simulink model "eTRU_prototype_2_old_perhabs_with_measurements"  (R2021b)
settings: Solver=daessc  StartTime=0.0  StopTime=5000  MaxStep=1  RelTol=1e-2  AbsTol=1e-2
PostLoadFcn:
  | eTRU_prototype_2_init
InitFcn:
  | eTRU_prototype_2_start_sim
StartFcn:
  | tic
StopFcn:
  | toc
  | PlotSimResults
values from neighbouring files (symbols this model uses):
  AirFlow = [0 0 0 0 0 0 0 0 0 0;      2205 1950 1701 1679 1297 658 0 0 0 0;      2989 2767 2610 2594 2410 2343 2274 1771 0 0;      3704 3545 3432 3422 3307 3266 3216 2958 2888 2215]    [EC_FanData.m]
  ambient_temp = 20    [eTRU_prototype_2_start_sim.m]
  asm = block.DialogPrm(1).Data    [msfcn_StaticASM.m]
  box_start_temp = 20    [eTRU_prototype_2_start_sim.m]
  cargo_start_temp = box_start_temp    (= 20)    [eTRU_prototype_2_start_sim.m]
  Power = [5 5 5 5 5 5 5 5 5 5;      185 203 227 226 229 230 231 237 239 247;      420 442 458 461 496 509 522 528 530 538;      764 811 844 846 880 892 905 969 987 989]    [EC_FanData.m]
  Pressure = LimitValue(Pressure + LimitValue(Error/dvdP, -0.1, 0.1), obj.PressureMin/100000, obj.PressureMax/100000)    [CoolPropPyWrapper.m]    (also in EC_FanData.m = [0,127,217,225,316,349,383,559,607,865])
  Speed = [0,1840,2450,3060]    [EC_FanData.m]
libraries: fl_lib x109, nesl_utility x82, simulink_extras x13, SimscapeFluids_lib x4
(part 2 of 3)

== system eTRU_prototype_2_old_perhabs_with_measurements/Evap_exv ==
  Vexp : Inport
  Gain3 : Gain  Gain=(0.007/2)^2*pi/100
  RefSensor : Subsystem
      settings: PortSchema="{\"entries\":[{\"content\":{\"sides\":[{\"content\":{\"connectorIds\":[\"LConn1\",\"Out1\"]},\"type\":\"ConnectorPlacement.EquallySpacedRectSide\",\"uuid\":\"384ca129-c08e-4242-8b56-38a57a5275bd\"},{\"content\":{\"connectorIds\":[\"RConn1\"],\"side\":\"RIGHT\"},\"type\":\"ConnectorPlacement.EquallySpacedRectSide\",\"uuid\":\"d8d27130-51db-4533-93b1-df7418a29f3a\"},{\"content\":{\"connectorIds\":[],\"side\":\"TOP\"},\"type\":\"ConnectorPlacement.EquallySpacedRectSide\",\"uuid\":\"67192aad-d15e-443e-8c24-a3a889184c8d\"},{\"content\":{\"connectorIds\":[],\"side\":\"BOTTOM\"},\"type\":\"ConnectorPlacement.EquallySpacedRectSide\",\"uuid\":\"18e5bc3a-5c8d-47f7-9803-91861ffb04f2\"}]},\"type\":\"ConnectorPlacement.EquallySpacedConnector\",\"uuid\":\"971e7a76-7cfc-4fb4-bbb6-a40c097b0bda\"}],\"packageUris\":[\"http://schema.mathworks.com/mf0/Connector/19700101\"],\"version\":\"1.0\"}"
  Simulink-PS Converter2 : nesl_utility/Simulink-PS Converter  PhysicalDomain=network_engine_domain  SubClassName=ps_input  LeftPortType=input  RightPortType=output  PseudoPeriodic=off  Frequencies=[]  NoiseDistribution=none  NoiseParameters=[]  Unit=m^2  AffineConversion=off  FilteringAndDerivatives=zero  SimscapeFilterOrder=1  InputFilterTimeConstant=0.001  UdotUserProvided=1
      settings: SourceProductBaseCode=PW,SS
  Transfer Fcn (with initial outputs) : simulink_extras/Additional Linear/Transfer Fcn (with initial outputs)  N=[1]  D="[1  1]"  Y0=0  U0=0
  Valve : fl_lib/Two-Phase Fluid/Elements/Variable Local Restriction (2P)  min_area=10e-10 mm^2  max_area=100 mm^2  area=(20/2)^2*pi mm^2  Cd=0.64  B_lam=0.999
      settings: SourceProductBaseCode=SS  InternalSimscapePortConfiguration="{\"Bottom\":[],\"Left\":[{\"id\":\"A\",\"label\":\"A\",\"type\":\"foundation.two_phase_fluid.two_phase_fluid\"},{\"id\":\"area_in\",\"label\":\"AR\",\"type\":\"input\"}],\"Right\":[{\"id\":\"B\",\"label\":\"B\",\"type\":\"foundation.two_phase_fluid.two_phase_fluid\"}],\"Top\":[]}"
  In : PMIOPort  Side=Left
  Out : PMIOPort  Port=2  Side=Right
  RefOutMeas : Outport
  wires:
  Gain3/1 -> Simulink-PS Converter2/1
  Vexp/1 -> Transfer Fcn (with initial outputs)/1
  Transfer Fcn (with initial outputs)/1 -> Gain3/1
  RefSensor/1(meas_out) -> RefOutMeas/1
  connections:
  Valve/LConn2 -- Simulink-PS Converter2/RConn1
  Valve/LConn1 -- In/RConn1
  Valve/RConn1 -- RefSensor/LConn1
  Out/RConn1 -- RefSensor/RConn1

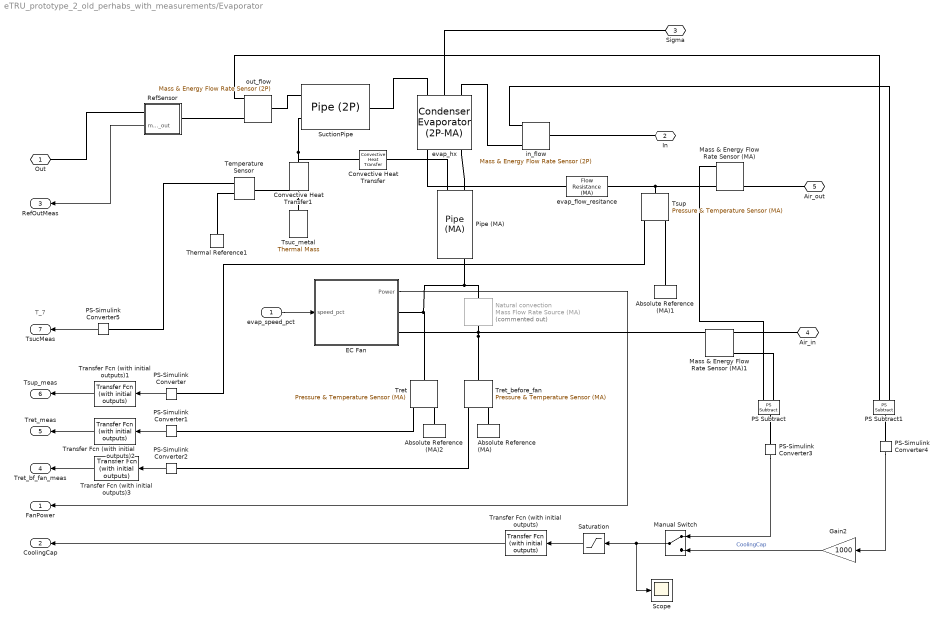
== system eTRU_prototype_2_old_perhabs_with_measurements/Evaporator ==
  note: T_7
  evap_speed_pct : Inport
  Absolute Reference (MA) : fl_lib/Moist Air/Elements/Absolute Reference (MA)
      settings: SourceProductBaseCode=SS
  Absolute Reference (MA)1 : fl_lib/Moist Air/Elements/Absolute Reference (MA)
      settings: SourceProductBaseCode=SS
  Absolute Reference (MA)2 : fl_lib/Moist Air/Elements/Absolute Reference (MA)
      settings: SourceProductBaseCode=SS
  Convective Heat Transfer : fl_lib/Thermal/Thermal Elements/Convective Heat Transfer  area=1 m^2  heat_tr_coeff=200 W/(m^2 * K)  T_specify=off  T_priority=None  T=0 K  T_nominal_specify=off  T_nominal_unit=K  T_nominal_value=1  Q_specify=off  Q_priority=None  Q=0 W  Q_nominal_specify=off  Q_nominal_unit=W  Q_nominal_value=1
  Convective Heat Transfer1 : fl_lib/Thermal/Thermal Elements/Convective Heat Transfer  area=1 m^2  heat_tr_coeff=100 W/(m^2 * K)  T_specify=off  T_priority=None  T=0 K  T_nominal_specify=off  T_nominal_unit=K  T_nominal_value=1  Q_specify=off  Q_priority=None  Q=0 W  Q_nominal_specify=off  Q_nominal_unit=W  Q_nominal_value=1
  EC Fan : Subsystem
      mask help:
      | Model of EC Fan with air flow and power consumption based on 2D table look-up.
      | Speed and pressure difference is used as table look-up input
      | The data is stored in the file EC_FanData.m that is loaded via model callback.
      | Full speed 100% is 3060 rpm
      |
      | Input:
      | Fan Speed [%] Speed reference
      | Pdiff [Pa]  pressure difference
      |
      | Output:
      | Power [Watt]Power consumption
      | Air_in, Air_out Simscape port for volumetric airflow rate
  Gain2 : Gain  Gain=1000
  Manual Switch : ManualSwitch
  Mass & Energy Flow Rate Sensor (MA) : fl_lib/Moist Air/Sensors/Mass & Energy Flow Rate Sensor (MA)
      settings: SourceProductBaseCode=SS  InternalSimscapePortConfiguration="{\"Bottom\":[],\"Left\":[{\"id\":\"A\",\"label\":\"A\",\"type\":\"foundation.moist_air.moist_air\"},{\"id\":\"Mw\",\"label\":\"Mw\",\"type\":\"output\"},{\"id\":\"Mg\",\"label\":\"Mg\",\"type\":\"output\"}],\"Right\":[{\"id\":\"B\",\"label\":\"B\",\"type\":\"foundation.moist_air.moist_air\"},{\"id\":\"M\",\"label\":\"M\",\"type\":\"output\"},{\"id\":\"PHI\",\"label\":\"Phi\",\"type\":\"output\"}],\"Top\":[]}"
  Mass & Energy Flow Rate Sensor (MA)1 : fl_lib/Moist Air/Sensors/Mass & Energy Flow Rate Sensor (MA)
      settings: SourceProductBaseCode=SS  InternalSimscapePortConfiguration="{\"Bottom\":[],\"Left\":[{\"id\":\"A\",\"label\":\"A\",\"type\":\"foundation.moist_air.moist_air\"},{\"id\":\"Mw\",\"label\":\"Mw\",\"type\":\"output\"},{\"id\":\"Mg\",\"label\":\"Mg\",\"type\":\"output\"}],\"Right\":[{\"id\":\"B\",\"label\":\"B\",\"type\":\"foundation.moist_air.moist_air\"},{\"id\":\"M\",\"label\":\"M\",\"type\":\"output\"},{\"id\":\"PHI\",\"label\":\"Phi\",\"type\":\"output\"}],\"Top\":[]}"
  Natural convection : fl_lib/Moist Air/Sources/Mass Flow Rate Source (MA)  Commented=on  power_spec=foundation.enum.power_spec.none  mass_flow=0 kg/s  area_A=1 m^2  area_B=1 m^2
      settings: SourceProductBaseCode=SS  InternalSimscapePortConfiguration="{\"Bottom\":[],\"Left\":[{\"id\":\"A\",\"label\":\"A\",\"type\":\"foundation.moist_air.moist_air\"}],\"Right\":[{\"id\":\"B\",\"label\":\"B\",\"type\":\"foundation.moist_air.moist_air\"}],\"Top\":[]}"
  PS Subtract : fl_lib/Physical Signals/Functions/PS Subtract
  PS Subtract1 : fl_lib/Physical Signals/Functions/PS Subtract
  PS-Simulink Converter{,1..5} (6 alike) : nesl_utility/PS-Simulink Converter  PhysicalDomain=network_engine_domain  SubClassName=ps_output  LeftPortType=input  RightPortType=output  PseudoPeriodic=off  Frequencies=[]  Unit=inherit  AffineConversion=off
      settings: SourceProductBaseCode=PW,SS
  Pipe (MA) : fl_lib/Moist Air/Elements/Pipe (MA)  length=1 m  area=1 m^2  Dh=1 m  length_add=0.1 m  roughness=15e-6 m  Re_lam=2000  Re_tur=4000  shape_factor=64  Nu_lam=3.66  RH_ws=1  time_constant=1e-3 s  moisture_trace_gas_source=foundation.enum.moisture_trace_gas_source.none  moisture_source_spec=foundation.enum.moisture_source_spec.vapor  moisture_mass_flow=0 kg/s  moisture_temperature_spec=foundation.enum.temperature_spec.atmospheric  moisture_temperature=293.15 K  trace_gas_mass_flow=0 kg/s  trace_gas_temperature_spec=foundation.enum.temperature_spec.atmospheric  trace_gas_temperature=293.15 K  p_I_specify=off  p_I_priority=High  p_I=0.101325 MPa  p_I_nominal_specify=off  p_I_nominal_unit=MPa  p_I_nominal_value=1  T_I_specify=off  T_I_priority=High  T_I=293.15 K  T_I_nominal_specify=off  T_I_nominal_unit=K  T_I_nominal_value=1  RH_I_specify=on  RH_I_priority=High  RH_I=0.5  RH_I_nominal_specify=off  RH_I_nominal_unit=1  RH_I_nominal_value=1  x_w_I_specify=off  x_w_I_priority=None  x_w_I=0  x_w_I_nominal_specify=off  x_w_I_nominal_unit=1  x_w_I_nominal_value=1  y_w_I_specify=off  y_w_I_priority=None  y_w_I=0  y_w_I_nominal_specify=off  y_w_I_nominal_unit=1  y_w_I_nominal_value=1  HR_I_specify=off  HR_I_priority=None  HR_I=0  HR_I_nominal_specify=off  HR_I_nominal_unit=1  HR_I_nominal_value=1  x_g_I_specify=off  x_g_I_priority=High  x_g_I=0  x_g_I_nominal_specify=off  x_g_I_nominal_unit=1  x_g_I_nominal_value=1  y_g_I_specify=off  y_g_I_priority=None  y_g_I=0  y_g_I_nominal_specify=off  y_g_I_nominal_unit=1  y_g_I_nominal_value=1
      settings: SourceProductBaseCode=SS
  RefSensor : Subsystem
  Saturation : Saturate  UpperLimit=20000  LowerLimit=-20000
  Scope : Scope
  SuctionPipe : fl_lib/Two-Phase Fluid/Elements/Pipe (2P)  length=1 m  area=0.02^2*pi m^2  Dh=0.02 m  length_add=0.1 m  roughness=15e-6 m  Re_lam=2000  Re_tur=4000  shape_factor=64  Nu_lam=3.66  inertia=simscape.enum.onoff.off  energy_spec=foundation.enum.energy_spec.quality  p_init=start_pressure_low bar  T_init=box_start_temp degC  x_init=1  alpha_init=0.1  h_init=1500 kJ/kg  u_init=1500 kJ/kg  mdot_init=0 kg/s  time_constant=0.1 s
      settings: SourceProductBaseCode=SS  InternalSimscapePortConfiguration="{\"Bottom\":[],\"Left\":[{\"id\":\"A\",\"label\":\"A\",\"type\":\"foundation.two_phase_fluid.two_phase_fluid\"},{\"id\":\"H\",\"label\":\"H\",\"type\":\"foundation.thermal.thermal\"}],\"Right\":[{\"id\":\"B\",\"label\":\"B\",\"type\":\"foundation.two_phase_fluid.two_phase_fluid\"}],\"Top\":[]}"
  Temperature Sensor : fl_lib/Thermal/Thermal Sensors/Temperature Sensor
  Thermal Reference1 : fl_lib/Thermal/Thermal Elements/Thermal Reference
  Transfer Fcn (with initial outputs) : simulink_extras/Additional Linear/Transfer Fcn (with initial outputs)  N=[0.1]  D=[1 0.1]  Y0=0  U0=0
  Transfer Fcn (with initial outputs)1 : simulink_extras/Additional Linear/Transfer Fcn (with initial outputs)  N=[0.1]  D="[1  0.1]"  Y0=box_start_temp+273.15  U0=box_start_temp+273.15
  Transfer Fcn (with initial outputs)2 : simulink_extras/Additional Linear/Transfer Fcn (with initial outputs)  N=[0.1]  D="[1  0.1]"  Y0=box_start_temp+273.15  U0=box_start_temp+273.15
  Transfer Fcn (with initial outputs)3 : simulink_extras/Additional Linear/Transfer Fcn (with initial outputs)  N=[0.1]  D="[1  0.1]"  Y0=box_start_temp+273.15  U0=box_start_temp+273.15
  Tret : fl_lib/Moist Air/Sensors/Pressure & Temperature Sensor (MA)
      settings: SourceProductBaseCode=SS  InternalSimscapePortConfiguration="{\"Bottom\":[],\"Left\":[{\"id\":\"A\",\"label\":\"A\",\"type\":\"foundation.moist_air.moist_air\"}],\"Right\":[{\"id\":\"B\",\"label\":\"B\",\"type\":\"foundation.moist_air.moist_air\"},{\"id\":\"P\",\"label\":\"P\",\"type\":\"output\"},{\"id\":\"T\",\"label\":\"T\",\"type\":\"output\"}],\"Top\":[]}"
  Tret_before_fan : fl_lib/Moist Air/Sensors/Pressure & Temperature Sensor (MA)
      settings: SourceProductBaseCode=SS  InternalSimscapePortConfiguration="{\"Bottom\":[],\"Left\":[{\"id\":\"A\",\"label\":\"A\",\"type\":\"foundation.moist_air.moist_air\"}],\"Right\":[{\"id\":\"B\",\"label\":\"B\",\"type\":\"foundation.moist_air.moist_air\"},{\"id\":\"P\",\"label\":\"P\",\"type\":\"output\"},{\"id\":\"T\",\"label\":\"T\",\"type\":\"output\"}],\"Top\":[]}"
  Tsuc_metal : fl_lib/Thermal/Thermal Elements/Thermal Mass  mass=0.5 kg  sp_heat=900 J/kg/K  T_specify=on  T_priority=None  T=box_start_temp degC  T_nominal_specify=off  T_nominal_unit=K  T_nominal_value=1  Q_specify=off  Q_priority=None  Q=0 W  Q_nominal_specify=off  Q_nominal_unit=W  Q_nominal_value=1
  Tsup : fl_lib/Moist Air/Sensors/Pressure & Temperature Sensor (MA)
      settings: SourceProductBaseCode=SS  InternalSimscapePortConfiguration="{\"Bottom\":[],\"Left\":[{\"id\":\"A\",\"label\":\"A\",\"type\":\"foundation.moist_air.moist_air\"}],\"Right\":[{\"id\":\"B\",\"label\":\"B\",\"type\":\"foundation.moist_air.moist_air\"},{\"id\":\"P\",\"label\":\"P\",\"type\":\"output\"},{\"id\":\"T\",\"label\":\"T\",\"type\":\"output\"}],\"Top\":[]}"
  evap_flow_resitance : fl_lib/Moist Air/Elements/Flow Resistance (MA)  delta_p_nominal=250 Pa  mdot_nominal=1 kg/s  rho_nominal=0 kg/m^3  area=1 m^2  laminar_fraction=1e-3
      settings: SourceProductBaseCode=SS
  evap_hx : SimscapeFluids_lib/Fluid Network Interfaces/Heat Exchangers/Condenser Evaporator (2P-MA)  flow_arrangement=fluids.interfaces.heat_exchangers.enum.FlowArrangement2PMA.Counter  cross_flow_arrangement=fluids.interfaces.heat_exchangers.enum.CrossFlowArrangement2PMA.UnmixedUnmixed  R_wall=0.1 K/kW  area_A1=0.02 m^2  area_B1=0.02 m^2  area_A2=1 m^2  area_B2=1 m^2  tube_num_2P=14  tube_length_2P=1.8*6 m  tube_cross_section_2P=fluids.interfaces.heat_exchangers.enum.TubeCrossSection.Circular  tube_diameter_2P=0.01 m  tube_width_2P=0.1 m  tube_height_2P=0.1 m  tube_inner_diameter_2P=0.05 m  tube_outer_diameter_2P=0.1 m  tube_flow_area_2P=0.01 m^2  tube_wetted_perimeter_2P=0.4 m  tube_heat_perimeter_2P=0.4 m  tube_pressure_loss_spec_2P=fluids.interfaces.heat_exchangers.enum.TubePressureLossSpec2P.Haaland  tube_loss_coeff_2P=10  tube_length_add_2P=0.5 m  tube_roughness_pressure_2P=0.001 m  tube_Re_lam_pressure_2P=2000  tube_Re_tur_pressure_2P=4000  tube_shape_factor_generic_2P=64  tube_heat_coeff_spec_2P=fluids.interfaces.heat_exchangers.enum.TubeHeatCoeffSpec2P.Colburn  tube_colburn_coeff_liq_2P=[.023, .8, .33]  tube_colburn_coeff_mix_2P=[.05, .8, .33]  tube_colburn_coeff_vap_2P=[.023, .8, .33]  tube_roughness_heat_2P=15e-6 m  tube_Re_lam_heat_2P=2000  tube_Re_tur_heat_2P=4000  tube_Nu_lam_generic_2P=3.66  fouling_factor_2P=0.1 K*m^2/kW  fin_area_2P=0.1 m^2  fin_efficiency_2P=0.5  energy_spec_2P=foundation.enum.energy_spec.quality  p_init_2P=start_pressure_low bar  T_init_2P=box_start_temp degC  x_init_2P=0.7  alpha_init_2P=0.5  h_init_2P=1500 kJ/kg  u_init_2P=1500 kJ/kg  flow_geometry_MA=fluids.interfaces.heat_exchangers.enum.FlowGeometryMA.AcrossTubeBank  tube_num_MA=1  tube_length_MA=5 m  tube_cross_section_MA=fluids.interfaces.heat_exchangers.enum.TubeCrossSection.Circular  tube_diameter_MA=0.1 m  tube_width_MA=0.1 m  tube_height_MA=0.1 m  tube_inner_diameter_MA=0.05 m  tube_outer_diameter_MA=0.1 m  tube_flow_area_MA=0.01 m^2  tube_wetted_perimeter_MA=0.4 m  tube_heat_perimeter_MA=0.4 m  tube_pressure_loss_spec_MA=fluids.interfaces.heat_exchangers.enum.TubePressureLossSpec.Haaland  tube_loss_coeff_MA=1  tube_length_add_MA=0.1 m  tube_roughness_pressure_MA=15e-6 m  tube_Re_lam_pressure_MA=2000  tube_Re_tur_pressure_MA=4000  tube_shape_factor_generic_MA=64  tube_heat_coeff_spec_MA=fluids.interfaces.heat_exchangers.enum.TubeHeatCoeffSpec.Gneilinski  tube_colburn_coeff_MA=[0.23, 0.8, 1 / 3]  tube_roughness_heat_MA=15e-6 m  tube_Re_lam_heat_MA=2000  tube_Re_tur_heat_MA=4000  tube_Nu_lam_generic_MA=3.66  bank_arrangement_MA=fluids.interfaces.heat_exchangers.enum.BankArrangement.Staggered  bank_num_rows_MA=6  bank_tubes_per_row_MA=14  bank_width_MA=0.3 m  bank_tube_diameter_MA=0.012 m  bank_longitudinal_pitch_MA=0.04 m  bank_transverse_pitch_MA=0.04 m  bank_pressure_loss_spec_MA=fluids.interfaces.heat_exchangers.enum.BankPressureLossSpec.Euler  bank_euler_MA=1  bank_heat_coeff_spec_MA=fluids.interfaces.heat_exchangers.enum.BankHeatCoeffSpec.Martin  bank_colburn_coeff_MA=[.27, .63, .36]  generic_flow_area_MA=0.1 m^2  generic_heat_area_MA=2 m^2  generic_volume_MA=1 m^3  generic_loss_coeff_MA=1  generic_colburn_coeff_MA=[0.23, 0.8, 1 / 3]  fouling_factor_MA=0.1 K*m^2/kW  fin_area_MA=50 m^2  fin_efficiency_MA=0.8  p_init_MA=0.101325 MPa  T_init_MA=box_start_temp degC  moisture_spec_MA=foundation.enum.moisture_spec.mole_fraction  RH_init_MA=0.5  x_w_init_MA=0.01  y_w_init_MA=0.01  HR_init_MA=0.01  trace_gas_spec_MA=foundation.enum.trace_gas_spec.mole_fraction  x_g_init_MA=0.001  y_g_init_MA=0.001  RH_ws_MA=1
      settings: SourceProductBaseCode=SH  InternalSimscapePortConfiguration="{\"Bottom\":[],\"Left\":[{\"id\":\"A1\",\"label\":\"A1\",\"type\":\"foundation.two_phase_fluid.two_phase_fluid\"},{\"id\":\"Z\",\"label\":\"Z\",\"type\":\"output\"},{\"id\":\"B1\",\"label\":\"B1\",\"type\":\"foundation.two_phase_fluid.two_phase_fluid\"}],\"Right\":[{\"id\":\"A2\",\"label\":\"A2\",\"type\":\"foundation.moist_air.moist_air\"},{\"id\":\"W\",\"label\":\"W\",\"type\":\"output\"},{\"id\":\"B2\",\"label\":\"B2\",\"type\":\"foundation.moist_air.moist_air\"}],\"Top\":[]}"
  in_flow : fl_lib/Two-Phase Fluid/Sensors/Mass & Energy Flow Rate Sensor (2P)
      settings: SourceProductBaseCode=SS  InternalSimscapePortConfiguration="{\"Bottom\":[],\"Left\":[{\"id\":\"A\",\"label\":\"A\",\"type\":\"foundation.two_phase_fluid.two_phase_fluid\"}],\"Right\":[{\"id\":\"B\",\"label\":\"B\",\"type\":\"foundation.two_phase_fluid.two_phase_fluid\"},{\"id\":\"M\",\"label\":\"M\",\"type\":\"output\"},{\"id\":\"PHI\",\"label\":\"Phi\",\"type\":\"output\"}],\"Top\":[]}"
  out_flow : fl_lib/Two-Phase Fluid/Sensors/Mass & Energy Flow Rate Sensor (2P)
      settings: SourceProductBaseCode=SS  InternalSimscapePortConfiguration="{\"Bottom\":[],\"Left\":[{\"id\":\"A\",\"label\":\"A\",\"type\":\"foundation.two_phase_fluid.two_phase_fluid\"}],\"Right\":[{\"id\":\"B\",\"label\":\"B\",\"type\":\"foundation.two_phase_fluid.two_phase_fluid\"},{\"id\":\"M\",\"label\":\"M\",\"type\":\"output\"},{\"id\":\"PHI\",\"label\":\"Phi\",\"type\":\"output\"}],\"Top\":[]}"
  Out : PMIOPort  Side=Left
  In : PMIOPort  Port=2  Side=Right
  Sigma : PMIOPort  Port=3  Side=Right
  Air_in : PMIOPort  Port=4  Side=Right
  Air_out : PMIOPort  Port=5  Side=Right
  FanPower : Outport
  CoolingCap : Outport  Port=2
  RefOutMeas : Outport  Port=3
  Tret_bf_fan_meas : Outport  Port=4
  Tret_meas : Outport  Port=5
  Tsup_meas : Outport  Port=6
  TsucMeas : Outport  Port=7
  wires:
  PS-Simulink Converter/1 -> Transfer Fcn (with initial outputs)1/1
  PS-Simulink Converter1/1 -> Transfer Fcn (with initial outputs)2/1
  PS-Simulink Converter2/1 -> Transfer Fcn (with initial outputs)3/1
  Transfer Fcn (with initial outputs)1/1 -> Tsup_meas/1
  Transfer Fcn (with initial outputs)3/1 -> Tret_bf_fan_meas/1
  Transfer Fcn (with initial outputs)2/1 -> Tret_meas/1
  evap_speed_pct/1 -> EC Fan/1(speed_pct)
  EC Fan/1(Power) -> FanPower/1
  Saturation/1 -> Transfer Fcn (with initial outputs)/1
  Transfer Fcn (with initial outputs)/1 -> CoolingCap/1
  Manual Switch/1 -> Scope/1, Saturation/1
  PS-Simulink Converter3/1 -> Manual Switch/1
  PS-Simulink Converter4/1 -> Gain2/1
  Gain2/1 -> Manual Switch/2  "CoolingCap"
  PS-Simulink Converter5/1 -> TsucMeas/1
  RefSensor/1(meas_out) -> RefOutMeas/1
  connections:
  Temperature Sensor/LConn1 -- Convective Heat Transfer1/RConn1 -- Tsuc_metal/LConn1
  Thermal Reference1/LConn1 -- Temperature Sensor/RConn1
  Temperature Sensor/RConn2 -- PS-Simulink Converter5/LConn1
  Tret_before_fan/LConn1 -- EC Fan/RConn2 -- Mass & Energy Flow Rate Sensor (MA)1/LConn1 -- Natural convection/LConn1
  evap_flow_resitance/RConn1 -- Mass & Energy Flow Rate Sensor (MA)/RConn1 -- Tsup/LConn1
  Absolute Reference (MA)1/LConn1 -- Tsup/RConn1
  Absolute Reference (MA)2/LConn1 -- Tret/RConn1
  EC Fan/RConn1 -- Pipe (MA)/RConn1 -- Natural convection/RConn1 -- Tret/LConn1
  Absolute Reference (MA)/LConn1 -- Tret_before_fan/RConn1
  Tsup/RConn3 -- PS-Simulink Converter/LConn1
  Tret/RConn3 -- PS-Simulink Converter1/LConn1
  Tret_before_fan/RConn3 -- PS-Simulink Converter2/LConn1
  evap_hx/LConn3 -- SuctionPipe/RConn1
  Sigma/RConn1 -- evap_hx/LConn2
  PS-Simulink Converter3/LConn1 -- PS Subtract/RConn1
  Mass & Energy Flow Rate Sensor (MA)1/RConn1 -- Air_in/RConn1
  Mass & Energy Flow Rate Sensor (MA)/LConn1 -- Air_out/RConn1
  Mass & Energy Flow Rate Sensor (MA)/RConn3 -- PS Subtract/LConn1
  Mass & Energy Flow Rate Sensor (MA)1/RConn3 -- PS Subtract/LConn2
  in_flow/RConn3 -- PS Subtract1/LConn2
  PS Subtract1/RConn1 -- PS-Simulink Converter4/LConn1
  out_flow/RConn3 -- PS Subtract1/LConn1
  out_flow/LConn1 -- SuctionPipe/LConn1
  evap_hx/LConn1 -- in_flow/RConn1
  In/RConn1 -- in_flow/LConn1
  RefSensor/LConn1 -- out_flow/RConn1
  Out/RConn1 -- RefSensor/RConn1
  Convective Heat Transfer/RConn1 -- Pipe (MA)/LConn2
  Convective Heat Transfer1/LConn1 -- SuctionPipe/LConn2 -- Convective Heat Transfer/LConn1
  Pipe (MA)/LConn1 -- evap_hx/RConn1
  evap_flow_resitance/LConn1 -- evap_hx/RConn3

== system eTRU_prototype_2_old_perhabs_with_measurements/FT_exv ==
  VFT : Inport
  Gain2 : Gain  Gain=(0.005/2)^2*pi/100*8
  RefSensor : Subsystem
      settings: PortSchema="{\"entries\":[{\"content\":{\"sides\":[{\"content\":{\"connectorIds\":[\"LConn1\"]},\"type\":\"ConnectorPlacement.EquallySpacedRectSide\",\"uuid\":\"384ca129-c08e-4242-8b56-38a57a5275bd\"},{\"content\":{\"connectorIds\":[\"RConn1\",\"Out1\"],\"side\":\"RIGHT\"},\"type\":\"ConnectorPlacement.EquallySpacedRectSide\",\"uuid\":\"d8d27130-51db-4533-93b1-df7418a29f3a\"},{\"content\":{\"connectorIds\":[],\"side\":\"TOP\"},\"type\":\"ConnectorPlacement.EquallySpacedRectSide\",\"uuid\":\"67192aad-d15e-443e-8c24-a3a889184c8d\"},{\"content\":{\"connectorIds\":[],\"side\":\"BOTTOM\"},\"type\":\"ConnectorPlacement.EquallySpacedRectSide\",\"uuid\":\"18e5bc3a-5c8d-47f7-9803-91861ffb04f2\"}]},\"type\":\"ConnectorPlacement.EquallySpacedConnector\",\"uuid\":\"971e7a76-7cfc-4fb4-bbb6-a40c097b0bda\"}],\"packageUris\":[\"http://schema.mathworks.com/mf0/Connector/19700101\"],\"version\":\"1.0\"}"
  Simulink-PS Converter3 : nesl_utility/Simulink-PS Converter  PhysicalDomain=network_engine_domain  SubClassName=ps_input  LeftPortType=input  RightPortType=output  PseudoPeriodic=off  Frequencies=[]  NoiseDistribution=none  NoiseParameters=[]  Unit=m^2  AffineConversion=off  FilteringAndDerivatives=zero  SimscapeFilterOrder=1  InputFilterTimeConstant=0.001  UdotUserProvided=1
      settings: SourceProductBaseCode=PW,SS
  Transfer Fcn (with initial outputs)1 : simulink_extras/Additional Linear/Transfer Fcn (with initial outputs)  N=[1]  D="[1  1]"  Y0=0  U0=0
  Valve : fl_lib/Two-Phase Fluid/Elements/Variable Local Restriction (2P)  min_area=10e-10 mm^2  max_area=100 mm^2  area=(20/2)^2*pi mm^2  Cd=0.64  B_lam=0.999
      settings: SourceProductBaseCode=SS  InternalSimscapePortConfiguration="{\"Bottom\":[],\"Left\":[{\"id\":\"A\",\"label\":\"A\",\"type\":\"foundation.two_phase_fluid.two_phase_fluid\"},{\"id\":\"area_in\",\"label\":\"AR\",\"type\":\"input\"}],\"Right\":[{\"id\":\"B\",\"label\":\"B\",\"type\":\"foundation.two_phase_fluid.two_phase_fluid\"}],\"Top\":[]}"
  In : PMIOPort  Side=Left
  Out : PMIOPort  Port=2  Side=Right
  RefOutMeas : Outport
  wires:
  VFT/1 -> Transfer Fcn (with initial outputs)1/1
  Gain2/1 -> Simulink-PS Converter3/1
  Transfer Fcn (with initial outputs)1/1 -> Gain2/1
  RefSensor/1(meas_out) -> RefOutMeas/1
  connections:
  Simulink-PS Converter3/RConn1 -- Valve/LConn2
  Valve/LConn1 -- In/RConn1
  Valve/RConn1 -- RefSensor/LConn1
  Out/RConn1 -- RefSensor/RConn1

== system eTRU_prototype_2_old_perhabs_with_measurements/Flash tank ==
  Cap (2P) : fl_lib/Two-Phase Fluid/Elements/Cap (2P)  p_specify=off  p_priority=None  p=0.101325 MPa  p_nominal_specify=off  p_nominal_unit=MPa  p_nominal_value=1  u_specify=off  u_priority=None  u=1.5e+3 kJ/kg  u_nominal_specify=off  u_nominal_unit=kJ/kg  u_nominal_value=1
      settings: SourceProductBaseCode=SS  InternalSimscapePortConfiguration="{\"Bottom\":[],\"Left\":[{\"id\":\"A\",\"label\":\"\",\"type\":\"foundation.two_phase_fluid.two_phase_fluid\"}],\"Right\":[],\"Top\":[]}"
  "FT heat transfer " : fl_lib/Thermal/Thermal Elements/Convective Heat Transfer  area=0.5 m^2  heat_tr_coeff=100 W/(m^2 * K)  T_specify=off  T_priority=None  T=0 K  T_nominal_specify=off  T_nominal_unit=K  T_nominal_value=1  Q_specify=off  Q_priority=None  Q=0 W  Q_nominal_specify=off  Q_nominal_unit=W  Q_nominal_value=1
  RefSensor : Subsystem
      settings: PortSchema="{\"entries\":[{\"content\":{\"sides\":[{\"content\":{\"connectorIds\":[\"LConn1\"]},\"type\":\"ConnectorPlacement.EquallySpacedRectSide\",\"uuid\":\"384ca129-c08e-4242-8b56-38a57a5275bd\"},{\"content\":{\"connectorIds\":[\"RConn1\",\"Out1\"],\"side\":\"RIGHT\"},\"type\":\"ConnectorPlacement.EquallySpacedRectSide\",\"uuid\":\"d8d27130-51db-4533-93b1-df7418a29f3a\"},{\"content\":{\"connectorIds\":[],\"side\":\"TOP\"},\"type\":\"ConnectorPlacement.EquallySpacedRectSide\",\"uuid\":\"67192aad-d15e-443e-8c24-a3a889184c8d\"},{\"content\":{\"connectorIds\":[],\"side\":\"BOTTOM\"},\"type\":\"ConnectorPlacement.EquallySpacedRectSide\",\"uuid\":\"18e5bc3a-5c8d-47f7-9803-91861ffb04f2\"}]},\"type\":\"ConnectorPlacement.EquallySpacedConnector\",\"uuid\":\"971e7a76-7cfc-4fb4-bbb6-a40c097b0bda\"}],\"packageUris\":[\"http://schema.mathworks.com/mf0/Connector/19700101\"],\"version\":\"1.0\"}"
  RefSensor1 : Subsystem
  Tank : SimscapeFluids_lib/Two-Phase Fluid/Tanks & Accumulators/Receiver Accumulator (2P)  volume=0.005 m^3  area_AV=0.01 m^2  area_BV=0.01 m^2  area_AL=0.01 m^2  area_BL=0.01 m^2  V_frac_error=simscape.enum.assert.action.warn  V_frac_min=0.05  V_frac_max=0.95  V_frac_smooth=0.05  p_crit_error=simscape.enum.assert.action.warn  hc_vap=20 W/(m^2*K)  hc_liq=100 W/(m^2*K)  surface_area=1 m^2  receiver_accumulator_energy_spec=fluids.two_phase_fluid.enum.receiver_accumulator_energy_spec.volume_fraction  p_init=start_pressure_im bar  T_init=im_start_temp degC  M_frac_init=0.5  V_frac_init=0.5  h_init=1500 kJ/kg  u_init=1500 kJ/kg  tau_vap_cond=0.1 s
      settings: SourceProductBaseCode=SH  InternalSimscapePortConfiguration="{\"Bottom\":[],\"Left\":[{\"id\":\"AV\",\"label\":\"AV\",\"type\":\"foundation.two_phase_fluid.two_phase_fluid\"},{\"id\":\"AL\",\"label\":\"AL\",\"type\":\"foundation.two_phase_fluid.two_phase_fluid\"},{\"id\":\"H\",\"label\":\"H\",\"type\":\"foundation.thermal.thermal\"}],\"Right\":[{\"id\":\"BV\",\"label\":\"BV\",\"type\":\"foundation.two_phase_fluid.two_phase_fluid\"},{\"id\":\"BL\",\"label\":\"BL\",\"type\":\"foundation.two_phase_fluid.two_phase_fluid\"},{\"id\":\"L\",\"label\":\"L\",\"type\":\"output\"}],\"Top\":[]}"
  Liquid in : PMIOPort  Side=Left
  Vapor out : PMIOPort  Port=2  Side=Left
  Liquid out : PMIOPort  Port=3  Side=Left
  Level : PMIOPort  Port=4  Side=Right
  H : PMIOPort  Port=5  Side=Right
  liq_out_meas : Outport
  vap_out_meas : Outport  Port=2
  wires:
  RefSensor/1(meas_out) -> vap_out_meas/1
  RefSensor1/1(meas_out) -> liq_out_meas/1
  connections:
  Liquid in/RConn1 -- Tank/LConn1
  H/RConn1 -- "FT heat transfer "/RConn1
  Tank/LConn2 -- Cap (2P)/LConn1
  Tank/RConn3 -- Level/RConn1
  "FT heat transfer "/LConn1 -- Tank/LConn3
  Tank/RConn1 -- RefSensor/LConn1
  RefSensor/RConn1 -- Vapor out/RConn1
  Tank/RConn2 -- RefSensor1/LConn1
  RefSensor1/RConn1 -- Liquid out/RConn1

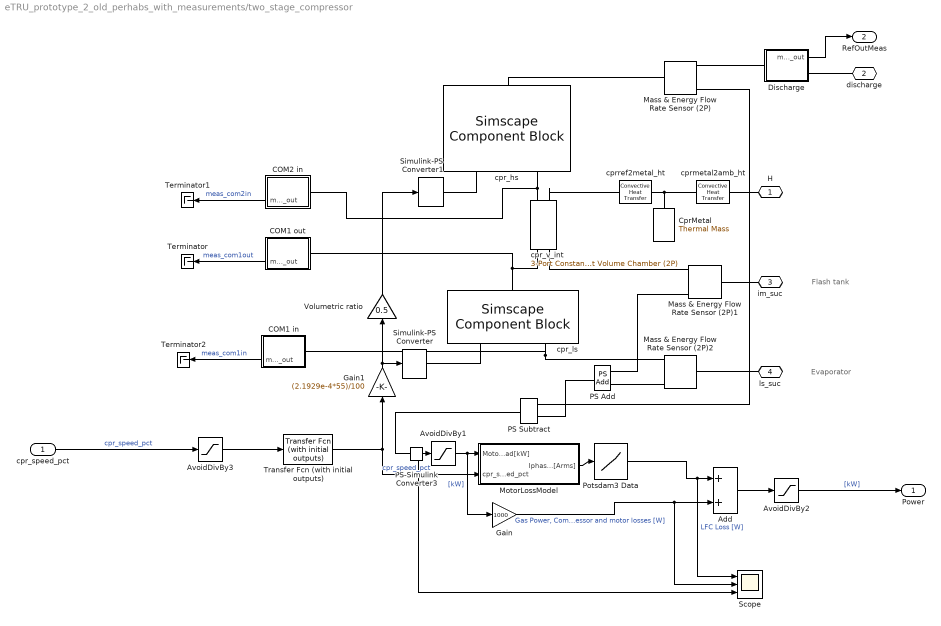
== system eTRU_prototype_2_old_perhabs_with_measurements/two_stage_compressor ==
  note: Evaporator
  note: Flash tank
  cpr_speed_pct : Inport
  Add : Sum
  AvoidDivBy1 : Saturate  UpperLimit=inf  LowerLimit=0
  AvoidDivBy2 : Saturate  UpperLimit=inf  LowerLimit=0
  AvoidDivBy3 : Saturate  UpperLimit=100  LowerLimit=0.01
  COM1 in : Subsystem
  COM1 out : Subsystem
  COM2 in : Subsystem
  CprMetal : fl_lib/Thermal/Thermal Elements/Thermal Mass  mass=50 kg  sp_heat=447 J/kg/K  T_specify=on  T_priority=Low  T=20 degC  T_nominal_specify=off  T_nominal_unit=K  T_nominal_value=1  Q_specify=off  Q_priority=None  Q=0 W  Q_nominal_specify=off  Q_nominal_unit=W  Q_nominal_value=1
  Discharge : Subsystem
  Gain : Gain  Gain=1000
  Gain1 : Gain  Gain=(2.1929e-4*55)/100
  Mass & Energy Flow Rate Sensor (2P) : fl_lib/Two-Phase Fluid/Sensors/Mass & Energy Flow Rate Sensor (2P)
      settings: SourceProductBaseCode=SS  InternalSimscapePortConfiguration="{\"Bottom\":[],\"Left\":[{\"id\":\"A\",\"label\":\"A\",\"type\":\"foundation.two_phase_fluid.two_phase_fluid\"}],\"Right\":[{\"id\":\"B\",\"label\":\"B\",\"type\":\"foundation.two_phase_fluid.two_phase_fluid\"},{\"id\":\"M\",\"label\":\"M\",\"type\":\"output\"},{\"id\":\"PHI\",\"label\":\"Phi\",\"type\":\"output\"}],\"Top\":[]}"
  Mass & Energy Flow Rate Sensor (2P)1 : fl_lib/Two-Phase Fluid/Sensors/Mass & Energy Flow Rate Sensor (2P)
      settings: SourceProductBaseCode=SS  InternalSimscapePortConfiguration="{\"Bottom\":[],\"Left\":[{\"id\":\"A\",\"label\":\"A\",\"type\":\"foundation.two_phase_fluid.two_phase_fluid\"}],\"Right\":[{\"id\":\"B\",\"label\":\"B\",\"type\":\"foundation.two_phase_fluid.two_phase_fluid\"},{\"id\":\"M\",\"label\":\"M\",\"type\":\"output\"},{\"id\":\"PHI\",\"label\":\"Phi\",\"type\":\"output\"}],\"Top\":[]}"
  Mass & Energy Flow Rate Sensor (2P)2 : fl_lib/Two-Phase Fluid/Sensors/Mass & Energy Flow Rate Sensor (2P)
      settings: SourceProductBaseCode=SS  InternalSimscapePortConfiguration="{\"Bottom\":[],\"Left\":[{\"id\":\"A\",\"label\":\"A\",\"type\":\"foundation.two_phase_fluid.two_phase_fluid\"}],\"Right\":[{\"id\":\"B\",\"label\":\"B\",\"type\":\"foundation.two_phase_fluid.two_phase_fluid\"},{\"id\":\"M\",\"label\":\"M\",\"type\":\"output\"},{\"id\":\"PHI\",\"label\":\"Phi\",\"type\":\"output\"}],\"Top\":[]}"
  MotorLossModel : Subsystem
  PS Add : fl_lib/Physical Signals/Functions/PS Add
  PS Subtract : fl_lib/Physical Signals/Functions/PS Subtract
  PS-Simulink Converter3 : nesl_utility/PS-Simulink Converter  PhysicalDomain=network_engine_domain  SubClassName=ps_output  LeftPortType=input  RightPortType=output  PseudoPeriodic=off  Frequencies=[]  Unit=inherit  AffineConversion=off
      settings: SourceProductBaseCode=PW,SS
  Potsdam3 Data : Lookup_n-D  NumberOfTableDimensions=1  BreakpointsForDimension1=[10 21]  BeginIndexSearchUsingPreviousIndexResult=on  Table=[66 178]  InternalRulePriority=Speed  RndMeth=Simplest  InputSameDT=on
  Scope : Scope  NumInputPorts=3
  Simulink-PS Converter : nesl_utility/Simulink-PS Converter  PhysicalDomain=network_engine_domain  SubClassName=ps_input  LeftPortType=input  RightPortType=output  PseudoPeriodic=off  Frequencies=[]  NoiseDistribution=none  NoiseParameters=[]  Unit=1  AffineConversion=off  FilteringAndDerivatives=zero  SimscapeFilterOrder=1  InputFilterTimeConstant=0.001  UdotUserProvided=1
      settings: SourceProductBaseCode=PW,SS
  Simulink-PS Converter1 : nesl_utility/Simulink-PS Converter  PhysicalDomain=network_engine_domain  SubClassName=ps_input  LeftPortType=input  RightPortType=output  PseudoPeriodic=off  Frequencies=[]  NoiseDistribution=none  NoiseParameters=[]  Unit=1  AffineConversion=off  FilteringAndDerivatives=zero  SimscapeFilterOrder=1  InputFilterTimeConstant=0.001  UdotUserProvided=1
      settings: SourceProductBaseCode=PW,SS
  Terminator : Terminator
  Terminator1 : Terminator
  Terminator2 : Terminator
  Transfer Fcn (with initial outputs) : simulink_extras/Additional Linear/Transfer Fcn (with initial outputs)  N=[1]  D="[1  1]"  Y0=0  U0=0
  Volumetric ratio : Gain  Gain=0.5
  cpr_hs : SimscapeComponentBlock  SourceFile=controlled_volumetric_flow_sink  ComponentPath=controlled_volumetric_flow_sink  ComponentVariants=controlled_volumetric_flow_sink  ComponentVariantNames=controlled_volumetric_flow_sink  ClassName=controlled_volumetric_flow_sink  SchemaVersion=1  power_spec=foundation.enum.power_spec.isentropic  isentropic_efficiency=0.65  area_A=0.01 m^2  area_B=0.01 m^2
      settings: CopyFcn=simscape.engine.sli.internal.componentblockcallback(gcbh,'COPY')  PreCopyFcn=simscape.engine.sli.internal.componentblockcallback(gcbh,'PRECOPY')  PreDeleteFcn=simscape.engine.sli.internal.componentblockcallback(gcbh,'PREDELETE')  InternalSimscapePortConfiguration="{\"Bottom\":[],\"Left\":[{\"id\":\"A\",\"label\":\"A\",\"type\":\"foundation.two_phase_fluid.two_phase_fluid\"},{\"id\":\"V\",\"label\":\"V\",\"type\":\"input\"}],\"Right\":[{\"id\":\"B\",\"label\":\"B\",\"type\":\"foundation.two_phase_fluid.two_phase_fluid\"}],\"Top\":[]}"
      mask Type: Controlled Volumetric Flow Rate Sink (2P)
  cpr_ls : SimscapeComponentBlock  SourceFile=controlled_volumetric_flow_sink  ComponentPath=controlled_volumetric_flow_sink  ComponentVariants=controlled_volumetric_flow_sink  ComponentVariantNames=controlled_volumetric_flow_sink  ClassName=controlled_volumetric_flow_sink  SchemaVersion=1  power_spec=foundation.enum.power_spec.isentropic  isentropic_efficiency=0.65  area_A=0.01 m^2  area_B=0.01 m^2
      settings: CopyFcn=simscape.engine.sli.internal.componentblockcallback(gcbh,'COPY')  PreCopyFcn=simscape.engine.sli.internal.componentblockcallback(gcbh,'PRECOPY')  PreDeleteFcn=simscape.engine.sli.internal.componentblockcallback(gcbh,'PREDELETE')  InternalSimscapePortConfiguration="{\"Bottom\":[],\"Left\":[{\"id\":\"A\",\"label\":\"A\",\"type\":\"foundation.two_phase_fluid.two_phase_fluid\"},{\"id\":\"V\",\"label\":\"V\",\"type\":\"input\"}],\"Right\":[{\"id\":\"B\",\"label\":\"B\",\"type\":\"foundation.two_phase_fluid.two_phase_fluid\"}],\"Top\":[]}"
      mask Type: Controlled Volumetric Flow Rate Sink (2P)
  cpr_v_int : fl_lib/Two-Phase Fluid/Elements/3-Port Constant Volume Chamber (2P)  volume=0.001 m^3  area_A=0.01 m^2  area_B=0.01 m^2  area_C=0.01 m^2  energy_spec=foundation.enum.energy_spec.quality  p_init=start_pressure_im bar  T_init=20 degC  x_init=1  alpha_init=0.5  h_init=1500 kJ/kg  u_init=1500 kJ/kg  time_constant=0.1 s
      settings: SourceProductBaseCode=SS  InternalSimscapePortConfiguration="{\"Bottom\":[],\"Left\":[{\"id\":\"A\",\"label\":\"A\",\"type\":\"foundation.two_phase_fluid.two_phase_fluid\"},{\"id\":\"H\",\"label\":\"H\",\"type\":\"foundation.thermal.thermal\"}],\"Right\":[{\"id\":\"B\",\"label\":\"B\",\"type\":\"foundation.two_phase_fluid.two_phase_fluid\"},{\"id\":\"C\",\"label\":\"C\",\"type\":\"foundation.two_phase_fluid.two_phase_fluid\"}],\"Top\":[]}"
  cprmetal2amb_ht : fl_lib/Thermal/Thermal Elements/Convective Heat Transfer  area=1 m^2  heat_tr_coeff=200 W/(m^2 * K)  T_specify=off  T_priority=None  T=0 K  T_nominal_specify=off  T_nominal_unit=K  T_nominal_value=1  Q_specify=off  Q_priority=None  Q=0 W  Q_nominal_specify=off  Q_nominal_unit=W  Q_nominal_value=1
  cprref2metal_ht : fl_lib/Thermal/Thermal Elements/Convective Heat Transfer  area=1 m^2  heat_tr_coeff=500 W/(m^2 * K)  T_specify=off  T_priority=None  T=0 K  T_nominal_specify=off  T_nominal_unit=K  T_nominal_value=1  Q_specify=off  Q_priority=None  Q=0 W  Q_nominal_specify=off  Q_nominal_unit=W  Q_nominal_value=1
  H : PMIOPort  Side=Left
  discharge : PMIOPort  Port=2  Side=Right
  im_suc : PMIOPort  Port=3  Side=Right
  ls_suc : PMIOPort  Port=4  Side=Right
  Power : Outport
  RefOutMeas : Outport  Port=2
  wires:
  Gain1/1 -> Volumetric ratio/1, Simulink-PS Converter/1
  Volumetric ratio/1 -> Simulink-PS Converter1/1
  cpr_speed_pct/1 -> AvoidDivBy3/1  "cpr_speed_pct"
  Transfer Fcn (with initial outputs)/1 -> MotorLossModel/2(cpr_speed_pct), Gain1/1  "cpr_speed_pct"
  Add/1 -> AvoidDivBy2/1
  Potsdam3 Data/1 -> Scope/1, Add/1  "LFC Loss [W]"
  MotorLossModel/1(Iphase[Arms]) -> Potsdam3 Data/1
  Gain/1 -> Scope/2, Add/2  "Gas Power, Compressor and motor losses [W]"
  AvoidDivBy1/1 -> Gain/1, MotorLossModel/1(MotorLoad[kW])  "[kW]"
  AvoidDivBy2/1 -> Power/1  "[kW]"
  PS-Simulink Converter3/1 -> AvoidDivBy1/1, Scope/3
  Discharge/1(meas_out) -> RefOutMeas/1
  AvoidDivBy3/1 -> Transfer Fcn (with initial outputs)/1
  COM1 out/1(meas_out) -> Terminator/1  "meas_com1out"
  COM2 in/1(meas_out) -> Terminator1/1  "meas_com2in"
  COM1 in/1(meas_out) -> Terminator2/1  "meas_com1in"
  connections:
  Simulink-PS Converter/RConn1 -- cpr_ls/LConn2
  Simulink-PS Converter1/RConn1 -- cpr_hs/LConn2
  cprmetal2amb_ht/RConn1 -- cprref2metal_ht/LConn1 -- CprMetal/LConn1
  cpr_v_int/LConn1 -- COM2 in/LConn1 -- cpr_hs/LConn1
  cpr_ls/RConn1 -- COM1 out/LConn1 -- cpr_v_int/RConn1
  cpr_v_int/LConn2 -- cprref2metal_ht/RConn1
  cprmetal2amb_ht/LConn1 -- H/RConn1
  Discharge/LConn1 -- Mass & Energy Flow Rate Sensor (2P)/RConn1
  Mass & Energy Flow Rate Sensor (2P)/LConn1 -- cpr_hs/RConn1
  PS Subtract/LConn1 -- Mass & Energy Flow Rate Sensor (2P)/RConn3
  Mass & Energy Flow Rate Sensor (2P)1/LConn1 -- im_suc/RConn1
  Mass & Energy Flow Rate Sensor (2P)1/RConn1 -- cpr_v_int/RConn2
  Mass & Energy Flow Rate Sensor (2P)1/RConn3 -- PS Add/LConn1
  Mass & Energy Flow Rate Sensor (2P)2/RConn1 -- COM1 in/LConn1 -- cpr_ls/LConn1
  PS Add/LConn2 -- Mass & Energy Flow Rate Sensor (2P)2/RConn3
  PS-Simulink Converter3/LConn1 -- PS Subtract/RConn1
  Mass & Energy Flow Rate Sensor (2P)2/LConn1 -- ls_suc/RConn1
  PS Subtract/LConn2 -- PS Add/RConn1
  Discharge/RConn1 -- discharge/RConn1

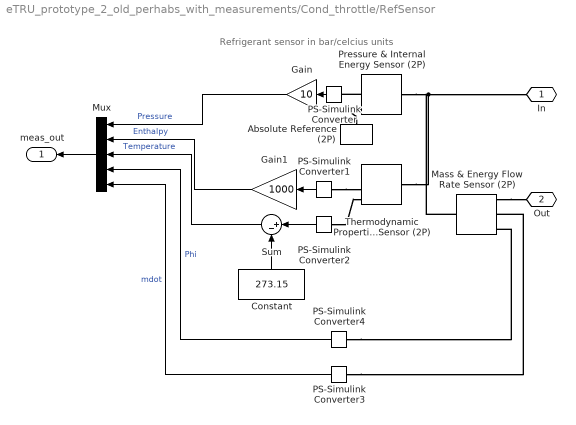
== system eTRU_prototype_2_old_perhabs_with_measurements/Cond_throttle/RefSensor ==
  note: Refrigerant sensor in bar/celcius units
  Absolute Reference (2P) : fl_lib/Two-Phase Fluid/Elements/Absolute Reference (2P)
      settings: SourceProductBaseCode=SS
  Constant : Constant  Value=273.15
  Gain : Gain  Gain=10
  Gain1 : Gain  Gain=1000
  Mass & Energy Flow Rate Sensor (2P) : fl_lib/Two-Phase Fluid/Sensors/Mass & Energy Flow Rate Sensor (2P)
      settings: SourceProductBaseCode=SS  InternalSimscapePortConfiguration="{\"Bottom\":[],\"Left\":[{\"id\":\"A\",\"label\":\"A\",\"type\":\"foundation.two_phase_fluid.two_phase_fluid\"}],\"Right\":[{\"id\":\"B\",\"label\":\"B\",\"type\":\"foundation.two_phase_fluid.two_phase_fluid\"},{\"id\":\"M\",\"label\":\"M\",\"type\":\"output\"},{\"id\":\"PHI\",\"label\":\"Phi\",\"type\":\"output\"}],\"Top\":[]}"
  Mux : Mux  Inputs=5
  PS-Simulink Converter{,1..4} (5 alike) : nesl_utility/PS-Simulink Converter  PhysicalDomain=network_engine_domain  SubClassName=ps_output  LeftPortType=input  RightPortType=output  PseudoPeriodic=off  Frequencies=[]  Unit=inherit  AffineConversion=off
      settings: SourceProductBaseCode=PW,SS
  Pressure & Internal Energy Sensor (2P) : fl_lib/Two-Phase Fluid/Sensors/Pressure & Internal Energy Sensor (2P)
      settings: SourceProductBaseCode=SS  InternalSimscapePortConfiguration="{\"Bottom\":[],\"Left\":[{\"id\":\"A\",\"label\":\"A\",\"type\":\"foundation.two_phase_fluid.two_phase_fluid\"}],\"Right\":[{\"id\":\"B\",\"label\":\"B\",\"type\":\"foundation.two_phase_fluid.two_phase_fluid\"},{\"id\":\"P\",\"label\":\"P\",\"type\":\"output\"},{\"id\":\"U\",\"label\":\"U\",\"type\":\"output\"}],\"Top\":[]}"
  Sum : Sum  Inputs=|+-
  Thermodynamic Properties Sensor (2P) : fl_lib/Two-Phase Fluid/Sensors/Thermodynamic Properties Sensor (2P)
      settings: SourceProductBaseCode=SS  InternalSimscapePortConfiguration="{\"Bottom\":[],\"Left\":[{\"id\":\"A\",\"label\":\"A\",\"type\":\"foundation.two_phase_fluid.two_phase_fluid\"}],\"Right\":[{\"id\":\"T\",\"label\":\"T\",\"type\":\"output\"},{\"id\":\"H\",\"label\":\"h\",\"type\":\"output\"},{\"id\":\"V\",\"label\":\"v\",\"type\":\"output\"},{\"id\":\"S\",\"label\":\"s\",\"type\":\"output\"}],\"Top\":[]}"
  In : PMIOPort  Side=Left
  Out : PMIOPort  Port=2  Side=Right
  meas_out : Outport
  wires:
  Sum/1 -> Mux/3  "Temperature"
  PS-Simulink Converter1/1 -> Gain1/1
  Gain/1 -> Mux/1  "Pressure"
  PS-Simulink Converter2/1 -> Sum/1
  Mux/1 -> meas_out/1
  PS-Simulink Converter/1 -> Gain/1
  Constant/1 -> Sum/2
  Gain1/1 -> Mux/2  "Enthalpy"
  PS-Simulink Converter4/1 -> Mux/4  "Phi"
  PS-Simulink Converter3/1 -> Mux/5  "mdot"
  connections:
  Pressure & Internal Energy Sensor (2P)/LConn1 -- In/RConn1 -- Thermodynamic Properties Sensor (2P)/LConn1 -- Mass & Energy Flow Rate Sensor (2P)/LConn1
  PS-Simulink Converter1/LConn1 -- Thermodynamic Properties Sensor (2P)/RConn2
  Pressure & Internal Energy Sensor (2P)/RConn1 -- Absolute Reference (2P)/LConn1
  Pressure & Internal Energy Sensor (2P)/RConn2 -- PS-Simulink Converter/LConn1
  PS-Simulink Converter2/LConn1 -- Thermodynamic Properties Sensor (2P)/RConn1
  Mass & Energy Flow Rate Sensor (2P)/RConn1 -- Out/RConn1
  PS-Simulink Converter4/LConn1 -- Mass & Energy Flow Rate Sensor (2P)/RConn3
  PS-Simulink Converter3/LConn1 -- Mass & Energy Flow Rate Sensor (2P)/RConn2

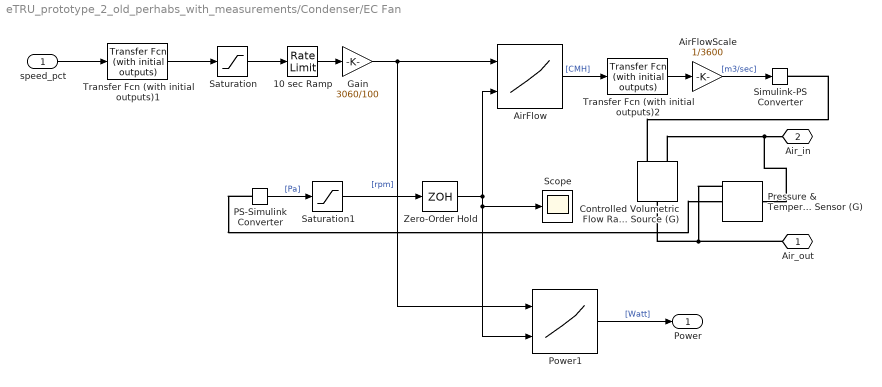
== system eTRU_prototype_2_old_perhabs_with_measurements/Condenser/EC Fan ==
  speed_pct : Inport
  10 sec Ramp : RateLimiter  RisingSlewLimit=300  FallingSlewLimit=-300  SampleTimeMode=inherited
  AirFlow : Lookup_n-D  BreakpointsForDimension1=Speed  BreakpointsForDimension2=Pressure  BeginIndexSearchUsingPreviousIndexResult=on  Table=AirFlow  InternalRulePriority=Speed  RndMeth=Simplest  InputSameDT=on
      settings: InputPortMap=u0,u1
  AirFlowScale : Gain  Gain=1/3600
  Controlled Volumetric Flow Rate Source (G) : fl_lib/Gas/Sources/Controlled Volumetric Flow Rate Source (G)  power_spec=foundation.enum.power_spec.isentropic  area_A=0.2 m^2  area_B=0.2 m^2
      settings: SourceProductBaseCode=SS  InternalSimscapePortConfiguration="{\"Bottom\":[],\"Left\":[{\"id\":\"A\",\"label\":\"A\",\"type\":\"foundation.gas.gas\"},{\"id\":\"V\",\"label\":\"V\",\"type\":\"input\"}],\"Right\":[{\"id\":\"B\",\"label\":\"B\",\"type\":\"foundation.gas.gas\"}],\"Top\":[]}"
  Gain : Gain  Gain=3060/100
  PS-Simulink Converter : nesl_utility/PS-Simulink Converter  PhysicalDomain=network_engine_domain  SubClassName=ps_output  LeftPortType=input  RightPortType=output  PseudoPeriodic=off  Frequencies=[]  Unit=inherit  AffineConversion=off
      settings: SourceProductBaseCode=PW,SS
  Power1 : Lookup_n-D  BreakpointsForDimension1=Speed  BreakpointsForDimension2=Pressure  BeginIndexSearchUsingPreviousIndexResult=on  Table=Power  InternalRulePriority=Speed  RndMeth=Simplest  InputSameDT=on
      settings: InputPortMap=u0,u1
  Pressure & Temperature Sensor (G) : fl_lib/Gas/Sensors/Pressure & Temperature Sensor (G)
      settings: SourceProductBaseCode=SS  InternalSimscapePortConfiguration="{\"Bottom\":[],\"Left\":[{\"id\":\"A\",\"label\":\"A\",\"type\":\"foundation.gas.gas\"}],\"Right\":[{\"id\":\"B\",\"label\":\"B\",\"type\":\"foundation.gas.gas\"},{\"id\":\"P\",\"label\":\"P\",\"type\":\"output\"},{\"id\":\"T\",\"label\":\"T\",\"type\":\"output\"}],\"Top\":[]}"
  Saturation : Saturate  UpperLimit=100  LowerLimit=0
  Saturation1 : Saturate  UpperLimit=865  LowerLimit=0
  Scope : Scope
  Simulink-PS Converter : nesl_utility/Simulink-PS Converter  PhysicalDomain=network_engine_domain  SubClassName=ps_input  LeftPortType=input  RightPortType=output  PseudoPeriodic=off  Frequencies=[]  NoiseDistribution=none  NoiseParameters=[]  Unit=1  AffineConversion=off  FilteringAndDerivatives=provide  SimscapeFilterOrder=1  InputFilterTimeConstant=0.001  UdotUserProvided=0
      settings: SourceProductBaseCode=PW,SS
  Transfer Fcn (with initial outputs)1 : simulink_extras/Additional Linear/Transfer Fcn (with initial outputs)  N=[1]  D="[1  1]"  Y0=0  U0=0
  Transfer Fcn (with initial outputs)2 : simulink_extras/Additional Linear/Transfer Fcn (with initial outputs)  N=[1]  D="[1  1]"  Y0=0  U0=0
  Zero-Order Hold : ZeroOrderHold  SampleTime=-1
  Air_out : PMIOPort  Side=Right
  Air_in : PMIOPort  Port=2  Side=Right
  Power : Outport
  wires:
  speed_pct/1 -> Transfer Fcn (with initial outputs)1/1
  Saturation/1 -> 10 sec Ramp/1
  10 sec Ramp/1 -> Gain/1
  Gain/1 -> Power1/1, AirFlow/1  "[rpm]"
  PS-Simulink Converter/1 -> Saturation1/1  "[Pa]"
  Saturation1/1 -> Zero-Order Hold/1
  Power1/1 -> Power/1  "[Watt]"
  AirFlow/1 -> Transfer Fcn (with initial outputs)2/1  "[CMH]"
  AirFlowScale/1 -> Simulink-PS Converter/1  "[m3/sec]"
  Transfer Fcn (with initial outputs)2/1 -> AirFlowScale/1
  Zero-Order Hold/1 -> AirFlow/2, Scope/1, Power1/2
  Transfer Fcn (with initial outputs)1/1 -> Saturation/1
  connections:
  Controlled Volumetric Flow Rate Source (G)/LConn1 -- Pressure & Temperature Sensor (G)/LConn1 -- Air_in/RConn1
  Controlled Volumetric Flow Rate Source (G)/LConn2 -- Simulink-PS Converter/RConn1
  PS-Simulink Converter/LConn1 -- Pressure & Temperature Sensor (G)/RConn2
  Air_out/RConn1 -- Pressure & Temperature Sensor (G)/RConn1 -- Controlled Volumetric Flow Rate Source (G)/RConn1

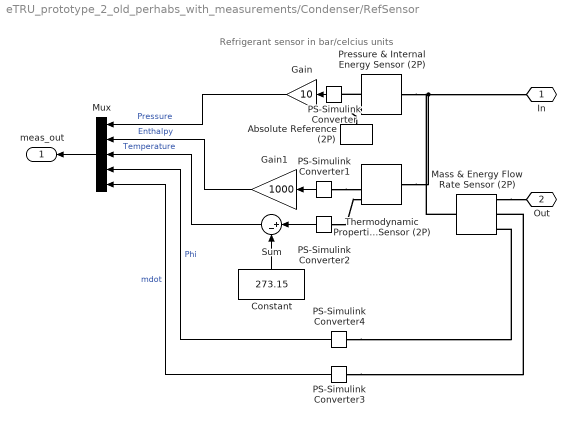
== system eTRU_prototype_2_old_perhabs_with_measurements/Condenser/RefSensor ==
  note: Refrigerant sensor in bar/celcius units
  Absolute Reference (2P) : fl_lib/Two-Phase Fluid/Elements/Absolute Reference (2P)
      settings: SourceProductBaseCode=SS
  Constant : Constant  Value=273.15
  Gain : Gain  Gain=10
  Gain1 : Gain  Gain=1000
  Mass & Energy Flow Rate Sensor (2P) : fl_lib/Two-Phase Fluid/Sensors/Mass & Energy Flow Rate Sensor (2P)
      settings: SourceProductBaseCode=SS  InternalSimscapePortConfiguration="{\"Bottom\":[],\"Left\":[{\"id\":\"A\",\"label\":\"A\",\"type\":\"foundation.two_phase_fluid.two_phase_fluid\"}],\"Right\":[{\"id\":\"B\",\"label\":\"B\",\"type\":\"foundation.two_phase_fluid.two_phase_fluid\"},{\"id\":\"M\",\"label\":\"M\",\"type\":\"output\"},{\"id\":\"PHI\",\"label\":\"Phi\",\"type\":\"output\"}],\"Top\":[]}"
  Mux : Mux  Inputs=5
  PS-Simulink Converter{,1..4} (5 alike) : nesl_utility/PS-Simulink Converter  PhysicalDomain=network_engine_domain  SubClassName=ps_output  LeftPortType=input  RightPortType=output  PseudoPeriodic=off  Frequencies=[]  Unit=inherit  AffineConversion=off
      settings: SourceProductBaseCode=PW,SS
  Pressure & Internal Energy Sensor (2P) : fl_lib/Two-Phase Fluid/Sensors/Pressure & Internal Energy Sensor (2P)
      settings: SourceProductBaseCode=SS  InternalSimscapePortConfiguration="{\"Bottom\":[],\"Left\":[{\"id\":\"A\",\"label\":\"A\",\"type\":\"foundation.two_phase_fluid.two_phase_fluid\"}],\"Right\":[{\"id\":\"B\",\"label\":\"B\",\"type\":\"foundation.two_phase_fluid.two_phase_fluid\"},{\"id\":\"P\",\"label\":\"P\",\"type\":\"output\"},{\"id\":\"U\",\"label\":\"U\",\"type\":\"output\"}],\"Top\":[]}"
  Sum : Sum  Inputs=|+-
  Thermodynamic Properties Sensor (2P) : fl_lib/Two-Phase Fluid/Sensors/Thermodynamic Properties Sensor (2P)
      settings: SourceProductBaseCode=SS  InternalSimscapePortConfiguration="{\"Bottom\":[],\"Left\":[{\"id\":\"A\",\"label\":\"A\",\"type\":\"foundation.two_phase_fluid.two_phase_fluid\"}],\"Right\":[{\"id\":\"T\",\"label\":\"T\",\"type\":\"output\"},{\"id\":\"H\",\"label\":\"h\",\"type\":\"output\"},{\"id\":\"V\",\"label\":\"v\",\"type\":\"output\"},{\"id\":\"S\",\"label\":\"s\",\"type\":\"output\"}],\"Top\":[]}"
  In : PMIOPort  Side=Left
  Out : PMIOPort  Port=2  Side=Right
  meas_out : Outport
  wires:
  Sum/1 -> Mux/3  "Temperature"
  PS-Simulink Converter1/1 -> Gain1/1
  Gain/1 -> Mux/1  "Pressure"
  PS-Simulink Converter2/1 -> Sum/1
  Mux/1 -> meas_out/1
  PS-Simulink Converter/1 -> Gain/1
  Constant/1 -> Sum/2
  Gain1/1 -> Mux/2  "Enthalpy"
  PS-Simulink Converter4/1 -> Mux/4  "Phi"
  PS-Simulink Converter3/1 -> Mux/5  "mdot"
  connections:
  Pressure & Internal Energy Sensor (2P)/LConn1 -- In/RConn1 -- Thermodynamic Properties Sensor (2P)/LConn1 -- Mass & Energy Flow Rate Sensor (2P)/LConn1
  PS-Simulink Converter1/LConn1 -- Thermodynamic Properties Sensor (2P)/RConn2
  Pressure & Internal Energy Sensor (2P)/RConn1 -- Absolute Reference (2P)/LConn1
  Pressure & Internal Energy Sensor (2P)/RConn2 -- PS-Simulink Converter/LConn1
  PS-Simulink Converter2/LConn1 -- Thermodynamic Properties Sensor (2P)/RConn1
  Mass & Energy Flow Rate Sensor (2P)/RConn1 -- Out/RConn1
  PS-Simulink Converter4/LConn1 -- Mass & Energy Flow Rate Sensor (2P)/RConn3
  PS-Simulink Converter3/LConn1 -- Mass & Energy Flow Rate Sensor (2P)/RConn2
